simulink model "UPSControl"  (R2025b)
settings: Solver=VariableStepAuto  StartTime=0.0  StopTime=10  FixedStep=Ts  RelTol=1e-3
PostLoadFcn:
  | DataCenterParam;
values from neighbouring files (symbols this model uses):
  generator = struct    [GeneratorParam.m]
  lineInductance = 1e-6    (= 1e-06)    [DataCenterParam.m]    (also in GridParam.m)
  lineResistance = 1e-3    (= 0.001)    [DataCenterParam.m]    (also in GridParam.m)
  loadPower = 5e6    (= 5000000)    [DataCenterParam.m]    (also in LVRT.m; RedundancyAnalysis.m = 10000000)
  machine = struct    [GeneratorParam.m]
  powerTau = 0.005    [DataCenterParam.m]
  Ts = 5e-5    (= 5e-05)    [DataCenterParam.m]    (also in GeneratorParam.m)
  utilizationFactor = 0.45    [DataCenterParam.m]    (also in RedundancyAnalysis.m)
undefined symbols (not defined in the file or in its folder): breaker, ctLimitDelayTime, DiscIntNeverNeededParam, ee_sli_rtmsupport, gcbh, grid, rack, ups
libraries: nesl_utility x96, fl_lib x96, eeGeneralControl x84, ee_lib x80, simulink x68, eeTransforms x30, nesl_utility_internal x16, eeSinusoidalMeasurementV2 x13, slpidlib x12, simulink_extras x12, datacenter_lib x5, batteryecm_lib x4
(part 9 of 13)

== system UPSControl/Server Load/UPS Units/Three UPS Parallel/UPS1/Rectifier/Transfer Control/PCC Voltage Flag ==
  u : Inport
  AND : Logic  IconShape=distinctive  AllPortsSameDT=off  OutDataTypeStr=boolean
  Abs : Abs  SaturateOnIntegerOverflow=off
  Add : Sum  Inputs=+-
  Compare To Constant : simulink/Logic and Bit Operations/Compare To Constant  relop=>  const=0.2  OutDataTypeStr=boolean
  Compare To Constant1 : simulink/Logic and Bit Operations/Compare To Constant  relop=>=  const=0.1  OutDataTypeStr=boolean
  Constant : Constant
  Data Type Conversion : DataTypeConversion  SaturateOnIntegerOverflow=off  RndMeth=Floor
  Data Type Conversion1 : DataTypeConversion  OutDataTypeStr=double  SaturateOnIntegerOverflow=off  RndMeth=Floor
  Discrete-Time Integrator : DiscreteIntegrator  IntegratorMethod=Integration: Backward Euler  ExternalReset=falling  SampleTime=ups.sampleTime  LimitOutput=on  UpperSaturationLimit=0.6  LowerSaturationLimit=0  ICPrevOutput=DiscIntNeverNeededParam  ICPrevScaledInput=DiscIntNeverNeededParam
  VFlag : Outport
  wires:
  AND/1 -> Data Type Conversion/1
  Compare To Constant/1 -> AND/2
  Discrete-Time Integrator/1 -> Compare To Constant/1
  Data Type Conversion/1 -> VFlag/1
  Data Type Conversion1/1 -> Discrete-Time Integrator/1, AND/1, Discrete-Time Integrator/2
  u/1 -> Add/1
  Constant/1 -> Add/2
  Add/1 -> Abs/1
  Compare To Constant1/1 -> Data Type Conversion1/1
  Abs/1 -> Compare To Constant1/1

== system UPSControl/Server Load/UPS Units/Three UPS Parallel/UPS1/Rectifier/Transfer Control/PCC Voltage Flag2 ==
  u : Inport
  AND : Logic  IconShape=distinctive  AllPortsSameDT=off  OutDataTypeStr=boolean
  Abs : Abs  SaturateOnIntegerOverflow=off
  Add : Sum  Inputs=+-
  Compare To Constant : simulink/Logic and Bit Operations/Compare To Constant  relop=>  const=0.15  OutDataTypeStr=boolean
  Compare To Constant1 : simulink/Logic and Bit Operations/Compare To Constant  relop=>=  const=0.9  OutDataTypeStr=boolean
  Constant : Constant
  Data Type Conversion : DataTypeConversion  SaturateOnIntegerOverflow=off  RndMeth=Floor
  Data Type Conversion1 : DataTypeConversion  OutDataTypeStr=double  SaturateOnIntegerOverflow=off  RndMeth=Floor
  Discrete-Time Integrator : DiscreteIntegrator  IntegratorMethod=Integration: Backward Euler  ExternalReset=falling  SampleTime=ups.sampleTime  LimitOutput=on  UpperSaturationLimit=4  LowerSaturationLimit=0  ICPrevOutput=DiscIntNeverNeededParam  ICPrevScaledInput=DiscIntNeverNeededParam
  VFlag : Outport
  wires:
  AND/1 -> Data Type Conversion/1
  Compare To Constant/1 -> AND/2
  Discrete-Time Integrator/1 -> Compare To Constant/1
  Data Type Conversion/1 -> VFlag/1
  Data Type Conversion1/1 -> Discrete-Time Integrator/1, AND/1, Discrete-Time Integrator/2
  u/1 -> Add/1
  Constant/1 -> Add/2
  Add/1 -> Abs/1
  Compare To Constant1/1 -> Data Type Conversion1/1
  Abs/1 -> Compare To Constant1/1

== system UPSControl/Server Load/UPS Units/Three UPS Parallel/UPS1/Rectifier/Transfer Control/PFC Current Flag ==
  u : Inport
  AND : Logic  IconShape=distinctive  AllPortsSameDT=off  OutDataTypeStr=boolean
  Compare To Constant : simulink/Logic and Bit Operations/Compare To Constant  relop=>  const=0.02  OutDataTypeStr=boolean
  Compare To Constant1 : simulink/Logic and Bit Operations/Compare To Constant  relop=<=  const=0.01  OutDataTypeStr=boolean
  Data Type Conversion : DataTypeConversion  SaturateOnIntegerOverflow=off  RndMeth=Floor
  Data Type Conversion1 : DataTypeConversion  OutDataTypeStr=double  SaturateOnIntegerOverflow=off  RndMeth=Floor
  Discrete-Time Integrator : DiscreteIntegrator  IntegratorMethod=Integration: Backward Euler  ExternalReset=falling  SampleTime=ups.sampleTime  LimitOutput=on  UpperSaturationLimit=0.04  LowerSaturationLimit=0  ICPrevOutput=DiscIntNeverNeededParam  ICPrevScaledInput=DiscIntNeverNeededParam
  Scope : Scope  NumInputPorts=2
      settings: ActiveDisplayYMinimum=-1  ActiveDisplayYMaximum=1  DataLoggingVariableName=ScopeData49
  Scope1 : Scope
      settings: ActiveDisplayYMinimum=-1  ActiveDisplayYMaximum=1  DataLoggingVariableName=ScopeData50
  IdFlag : Outport
  wires:
  AND/1 -> Data Type Conversion/1
  Compare To Constant1/1 -> Data Type Conversion1/1
  Compare To Constant/1 -> Scope/2, AND/2
  u/1 -> Compare To Constant1/1
  Discrete-Time Integrator/1 -> Scope1/1, Compare To Constant/1
  Data Type Conversion/1 -> IdFlag/1
  Data Type Conversion1/1 -> Scope/1, Discrete-Time Integrator/1, AND/1, Discrete-Time Integrator/2

== system UPSControl/Server Load/UPS Units/Three UPS Parallel/UPS2/DC-Link/BESS/DC-DC Converter Controller ==
  Voref : Inport
  Vo : Inport  Port=2
  vBatt : Inport  Port=3
  iPFC : Inport  Port=4
  iCharge : Inport  Port=5
  iBatt : Inport  Port=6
  vPCC : Inport  Port=7
  Breaker : Inport  Port=8
  Current Reference Generator : Subsystem
  Gain : Gain  Gain=iBatt
  Mode Control : Subsystem
  Saturation : Saturate  UpperLimit=iBatt  LowerLimit=-iBatt
  Simulink-PS Converter : nesl_utility/Simulink-PS Converter  PhysicalDomain=network_engine_domain  SubClassName=ps_input  LeftPortType=input  RightPortType=output  PseudoPeriodic=off  Frequencies=[]  NoiseDistribution=none  NoiseParameters=[]  Unit=1  AffineConversion=off  FilteringAndDerivatives=provide  SimscapeFilterOrder=1  InputFilterTimeConstant=0.001  UdotUserProvided=0
  Terminator1 : Terminator
  mod : PMIOPort  Side=Right
  wires:
  Gain/1 -> Saturation/1
  iPFC/1 -> Mode Control/1(iPFC)
  vBatt/1 -> Mode Control/3(vBatt)
  Current Reference Generator/1(i) -> Gain/1
  Mode Control/1(DischargeFlag) -> Current Reference Generator/2(DischargeFlag)
  Saturation/1 -> Simulink-PS Converter/1
  iBatt/1 -> Mode Control/7(iBatt)
  vPCC/1 -> Mode Control/4(vPCC)
  Breaker/1 -> Mode Control/5(Breaker)
  iCharge/1 -> Mode Control/6(iCharg)
  Vo/1 -> Mode Control/2(Vdc)
  Mode Control/3(iRef) -> Current Reference Generator/4(I)
  Mode Control/5(Mode) -> Terminator1/1
  Voref/1 -> Current Reference Generator/1(VoRef)
  Mode Control/2(vOut) -> Current Reference Generator/3(Vo)
  Mode Control/4(droopMode) -> Current Reference Generator/5(Mode)
  connections:
  mod/RConn1 -- Simulink-PS Converter/RConn1

== system UPSControl/Server Load/UPS Units/Three UPS Parallel/UPS2/Inverter/Filter & Measurements/PLL & Measurements ==
  V : Inport
  I : Inport  Port=2
  Measurement1 : Subsystem
  Measurement2 : Subsystem
  Subsystem : Subsystem
  Out Bus Element : Outport  PortName=VIbus  Element=Vq
  Out Bus Element1 : Outport  PortName=VIbus  Element=Vd
  Out Bus Element2 : Outport  PortName=VIbus  Element=Freq
  Out Bus Element3 : Outport  PortName=VIbus  Element=Theta
  Out Bus Element4 : Outport  PortName=VIbus  Element=Vmag
  Out Bus Element5 : Outport  PortName=VIbus  Element=Iq
  Out Bus Element6 : Outport  PortName=VIbus  Element=Id
  Out Bus Element7 : Outport  PortName=VIbus  Element=Iabc
  Out Bus Element8 : Outport  PortName=VIbus  Element=Vabc
  wires:
  Subsystem/6(Id1) -> Out Bus Element6/1
  Subsystem/7(Iq1) -> Out Bus Element5/1
  Measurement1/1(Vg) -> Subsystem/2(Iabc), Out Bus Element7/1
  I/1 -> Measurement1/1(u)
  Subsystem/1(mag) -> Out Bus Element4/1
  Measurement2/1(Vg) -> Subsystem/1(Vabc), Out Bus Element8/1
  Subsystem/4(Vd) -> Out Bus Element1/1
  Subsystem/3(angle) -> Out Bus Element3/1
  Subsystem/5(Vq) -> Out Bus Element/1
  Subsystem/2(freq) -> Out Bus Element2/1
  V/1 -> Measurement2/1(u)

== system UPSControl/Server Load/UPS Units/Three UPS Parallel/UPS2/Inverter/Inverter Controller/Current Limiter ==
  BusElementIn : Inport  PortName=VI  Element=Id
  BusElementIn1 : Inport  PortName=VI  Element=Iq
  Vd : Inport  Port=2
  Vq : Inport  Port=3
  Add : Sum  Inputs=+-
  Add1 : Sum  Inputs=+-
  Current Limiter : Subsystem  Variant=on  VariantControlMode=label  VariantControl=Choice  LabelModeActiveChoice=Virtual Impedance
  VdRef : Outport
  VqRef : Outport  Port=2
  Idmax : Outport  Port=3
  Iqmax : Outport  Port=4
  wires:
  BusElementIn/1 -> Current Limiter/1(Igd)
  BusElementIn1/1 -> Current Limiter/2(Igq)
  Current Limiter/3(Idmax) -> Idmax/1
  Current Limiter/4(Iqmax) -> Iqmax/1
  Current Limiter/1(delVd) -> Add/2
  Vd/1 -> Add/1
  Add1/1 -> VqRef/1
  Current Limiter/2(delVq) -> Add1/2
  Vq/1 -> Add1/1
  Add/1 -> VdRef/1

== system UPSControl/Server Load/UPS Units/Three UPS Parallel/UPS2/Inverter/Inverter Controller/Droop Control ==
  note: Frequency difference power
  note: Vs-delV
  BusElementIn : Inport  PortName=Power  Element=activePower
  BusElementIn1 : Inport  PortName=Power  Element=reactivePower
  Add : Sum  Inputs=+-
  Constant1 : Constant  Value=powerFreq*2*pi
  Constant3 : Constant
  Constant4 : Constant  Value=0
  Constant5 : Constant  Value=pi/2
  Gain1 : Gain  Gain=vDroop
  Gain6 : Gain  Gain=fDroop
  Integrator with Wrapped State (Discrete or Continuous) : eeGeneralControl/Integrator with Wrapped State (Discrete or Continuous)  LabelModeActiveChoice=Discrete  WrappedStateUpperValue=2*pi  WrappedStateLowerValue=0  x0=0  Ts=Ts
  Low-Pass Filter (Discrete or Continuous) : eeGeneralControl/Low-Pass Filter (Discrete or Continuous)  K=1  T=0.01  B=inf  A=-inf  init_option=Inherited from block input  x0=0  Ts=-1
  Low-Pass Filter (Discrete or Continuous)1 : eeGeneralControl/Low-Pass Filter (Discrete or Continuous)  K=1  T=0.01  B=inf  A=-inf  init_option=Inherited from block input  x0=0  Ts=-1
  Saturation : Saturate  UpperLimit=1.5  LowerLimit=0.9
  Scope : Scope
      settings: ActiveDisplayYMinimum=1.0057772633115749  ActiveDisplayYMaximum=1.0057796201435223  DataLoggingVariableName=ScopeData3  DataLoggingSaveFormat=Array
  Scope1 : Scope
      settings: ActiveDisplayYMinimum=-1  ActiveDisplayYMaximum=1  DataLoggingVariableName=ScopeData4
  Scope3 : Scope  NumInputPorts=2
      settings: ActiveDisplayYMinimum=-1  ActiveDisplayYMaximum=1  DataLoggingVariableName=ScopeData6  DataLoggingSaveFormat=Array
  Scope4 : Scope  NumInputPorts=2
      settings: ActiveDisplayYMinimum=-1  ActiveDisplayYMaximum=1  DataLoggingVariableName=ScopeData23
  Sum : Sum  Inputs=|++
  Sum1 : Sum  Inputs=|++
  Vdref : Outport
  Vqref : Outport  Port=2
  omega : Outport  Port=3
  Theta : Outport  Port=4
  wires:
  Low-Pass Filter (Discrete or Continuous)/1 -> Gain1/1
  Sum/1 -> Scope4/2, Integrator with Wrapped State (Discrete or Continuous)/1, omega/1
  Gain1/1 -> Sum1/2, Scope3/1
  Sum1/1 -> Scope3/2, Saturation/1  "V"
  Constant5/1 -> Add/2
  Constant3/1 -> Sum1/1
  Saturation/1 -> Scope/1, Vdref/1
  Integrator with Wrapped State (Discrete or Continuous)/1 -> Add/1
  Constant1/1 -> Sum/1
  Add/1 -> Scope1/1, Theta/1
  Gain6/1 -> Scope4/1, Sum/2
  Low-Pass Filter (Discrete or Continuous)1/1 -> Gain6/1
  BusElementIn/1 -> Low-Pass Filter (Discrete or Continuous)1/1
  Constant4/1 -> Vqref/1
  BusElementIn1/1 -> Low-Pass Filter (Discrete or Continuous)/1

== system UPSControl/Server Load/UPS Units/Three UPS Parallel/UPS2/Inverter/Inverter Controller/VoltageCurrentControl ==
  BusElementIn : Inport  PortName=measure  Element=Vq
  BusElementIn1 : Inport  PortName=measure  Element=Vd
  BusElementIn2 : Inport  PortName=measure  Element=Iq
  BusElementIn3 : Inport  PortName=measure  Element=Id
  Vdref : Inport  Port=2
  Vqref : Inport  Port=3
  Idmax : Inport  Port=4
  Iqmax : Inport  Port=5
  w : Inport  Port=6
  Angle : Inport  Port=7
  Controller : Subsystem
  Modulation Signal : Subsystem
  mabc : Outport
  wires:
  Vdref/1 -> Controller/2(Vdref)
  Controller/1(Vd) -> Modulation Signal/1(Vd)
  Modulation Signal/1(mabc) -> mabc/1
  Controller/2(Vq) -> Modulation Signal/2(Vq)
  w/1 -> Controller/1(Angfreq)
  Angle/1 -> Modulation Signal/3(Angle)
  BusElementIn/1 -> Controller/5(Vsq)
  BusElementIn1/1 -> Controller/4(Vsd)
  BusElementIn2/1 -> Controller/7(Iq)
  BusElementIn3/1 -> Controller/6(Id)
  Vqref/1 -> Controller/3(Vqref)
  Idmax/1 -> Controller/8(IqMax)
  Iqmax/1 -> Controller/9(IdMax)

== system UPSControl/Server Load/UPS Units/Three UPS Parallel/UPS2/Rectifier/Filter & AC measurements/Current ==
  Isabc : Inport
  Demux : Demux  Outputs=3
  Mux : Mux  Inputs=3
  Unit Delay : UnitDelay  SampleTime=-1
  Iabc : Outport
  wires:
  Mux/1 -> Iabc/1
  Unit Delay/1 -> Demux/1
  Isabc/1 -> Unit Delay/1
  Demux/1 -> Mux/1
  Demux/2 -> Mux/2
  Demux/3 -> Mux/3

== system UPSControl/Server Load/UPS Units/Three UPS Parallel/UPS2/Rectifier/Filter & AC measurements/PLL ==
  Iabc : Inport
  V : Inport  Port=2
  Constant1 : Constant  Value=pi/2  SampleTime=Ts
  Data Type Conversion Inherited : simulink/Signal Attributes/Data Type Conversion Inherited  ConvertRealWorld=Real World Value  DoSatur=off
  Demux : Demux  Outputs=3
  Park Transform : eeTransforms/Park Transform  AxisAlignment=D-axis  PowerInvariant=off
  "Sinusoidal Measurement (PLL, Three-Phase)" : eeSinusoidalMeasurementV2/Sinusoidal Measurement (PLL, Three-Phase)  InputFilter=on  InputNormalization=off  Kp_LF=ups.AFE.kpPLL  Ki_LF=ups.AFE.kiPLL  F0=frequency  Theta0=0  Ts=Ts
  Sum : Sum  Inputs=|+-
  Terminator : Terminator
  Terminator2 : Terminator
  Id : Outport
  freq : Outport  Port=2
  mag : Outport  Port=3
  wires:
  Data Type Conversion Inherited/1 -> Sum/2
  Constant1/1 -> Data Type Conversion Inherited/2
  V/1 -> "Sinusoidal Measurement (PLL, Three-Phase)"/1
  "Sinusoidal Measurement (PLL, Three-Phase)"/2 -> Sum/1, Data Type Conversion Inherited/1
  Park Transform/1 -> Demux/1
  Demux/3 -> Terminator/1
  Sum/1 -> Park Transform/2
  Demux/1 -> Id/1
  "Sinusoidal Measurement (PLL, Three-Phase)"/1 -> freq/1
  Iabc/1 -> Park Transform/1
  Demux/2 -> Terminator2/1
  "Sinusoidal Measurement (PLL, Three-Phase)"/3 -> mag/1

== system UPSControl/Server Load/UPS Units/Three UPS Parallel/UPS2/Rectifier/Filter & AC measurements/Voltage ==
  Vsabc : Inport
  Demux1 : Demux  Outputs=3
  Mux1 : Mux  Inputs=3
  Unit Delay : UnitDelay  SampleTime=-1
  Vabc : Outport
  wires:
  Mux1/1 -> Vabc/1
  Unit Delay/1 -> Demux1/1
  Vsabc/1 -> Unit Delay/1
  Demux1/1 -> Mux1/1
  Demux1/2 -> Mux1/2
  Demux1/3 -> Mux1/3

== system UPSControl/Server Load/UPS Units/Three UPS Parallel/UPS2/Rectifier/PFC Rectifier Controller/Current Controller ==
  idRef : Inport
  iqRef : Inport  Port=2
  theta : Inport  Port=3
  vd : Inport  Port=4
  vq : Inport  Port=5
  iabc(PU) : Inport  Port=6
  Reset : Inport  Port=7
  Demux1 : Demux  Outputs=3
  Id and Iq Controller : Subsystem
  Inverse Park Transform : eeTransforms/Inverse Park Transform  AxisAlignment=D-axis  PowerInvariant=off
  Park Transform : eeTransforms/Park Transform  AxisAlignment=D-axis  PowerInvariant=off
  Saturation : Saturate  UpperLimit=1.5  LowerLimit=-1.5
  Terminator1 : Terminator
  vabcRef : Outport
  IdCntrlError : Outport  Port=2
  IqCntrlError : Outport  Port=3
  wires:
  Id and Iq Controller/2(IdCntrlError) -> IdCntrlError/1
  Id and Iq Controller/3(IqCntrlError) -> IqCntrlError/1
  Id and Iq Controller/1(vdqoRef) -> Inverse Park Transform/1
  vq/1 -> Id and Iq Controller/6(vq)
  Demux1/2 -> Id and Iq Controller/4(iqSens)  "iqSens"
  iqRef/1 -> Id and Iq Controller/2(iqRef)
  Demux1/1 -> Id and Iq Controller/3(IdSens)  "IdSens"
  idRef/1 -> Id and Iq Controller/1(idRef)
  vd/1 -> Id and Iq Controller/5(vd)
  Inverse Park Transform/1 -> Saturation/1
  iabc(PU)/1 -> Park Transform/1
  theta/1 -> Park Transform/2, Inverse Park Transform/2
  Demux1/3 -> Terminator1/1
  Park Transform/1 -> Demux1/1
  Saturation/1 -> vabcRef/1
  Reset/1 -> Id and Iq Controller/7(Reset)

== system UPSControl/Server Load/UPS Units/Three UPS Parallel/UPS2/Rectifier/PFC Rectifier Controller/DC Voltage Controller and Current Reference ==
  qRef : Inport
  vPeak : Inport  Port=2
  vdcRef : Inport  Port=3
  VdcSens : Inport  Port=4
  Reset : Inport  Port=5
  Constant : Constant  SampleTime=Ts
  Data Type Conversion Inherited : simulink/Signal Attributes/Data Type Conversion Inherited  ConvertRealWorld=Real World Value  DoSatur=off
  Gain : Gain  Gain=-1
  Iq Reference : Subsystem
  Switch : Switch  Criteria=u2 > Threshold  SaturateOnIntegerOverflow=off  InputSameDT=off
  Voltage Controller : Subsystem
  idRef : Outport
  iqRef : Outport  Port=2
  wires:
  Constant/1 -> Data Type Conversion Inherited/2
  Data Type Conversion Inherited/1 -> Switch/3
  Gain/1 -> iqRef/1
  qRef/1 -> Iq Reference/2(Q_ref)
  Voltage Controller/1(Id) -> idRef/1
  vdcRef/1 -> Voltage Controller/1(Vdcref)
  VdcSens/1 -> Voltage Controller/2(Vdcmeas)
  Iq Reference/1(iq_ref) -> Gain/1
  vPeak/1 -> Switch/2, Switch/1, Data Type Conversion Inherited/1
  Switch/1 -> Iq Reference/1(V_mag)
  Reset/1 -> Voltage Controller/3(Reset)

== system UPSControl/Server Load/UPS Units/Three UPS Parallel/UPS2/Rectifier/PFC Rectifier Controller/PLL ==
  V : Inport
  Constant1 : Constant  Value=pi/2  SampleTime=Ts
  Data Type Conversion Inherited : simulink/Signal Attributes/Data Type Conversion Inherited  ConvertRealWorld=Real World Value  DoSatur=off
  Demux : Demux  Outputs=3
  Park Transform : eeTransforms/Park Transform  AxisAlignment=D-axis  PowerInvariant=off
  "Sinusoidal Measurement (PLL, Three-Phase)" : eeSinusoidalMeasurementV2/Sinusoidal Measurement (PLL, Three-Phase)  InputFilter=on  InputNormalization=off  Kp_LF=KpPLL  Ki_LF=KiPLL  F0=Freq  Theta0=0  Ts=Ts
  Sum : Sum  Inputs=|+-
  Terminator : Terminator
  Terminator1 : Terminator
  theta : Outport
  Vd : Outport  Port=2
  Vq : Outport  Port=3
  mag : Outport  Port=4
  wires:
  Data Type Conversion Inherited/1 -> Sum/2
  Constant1/1 -> Data Type Conversion Inherited/2
  V/1 -> Park Transform/1, "Sinusoidal Measurement (PLL, Three-Phase)"/1
  "Sinusoidal Measurement (PLL, Three-Phase)"/2 -> Sum/1, Data Type Conversion Inherited/1
  Park Transform/1 -> Demux/1
  Demux/3 -> Terminator/1
  "Sinusoidal Measurement (PLL, Three-Phase)"/3 -> mag/1
  Sum/1 -> Park Transform/2, theta/1
  Demux/2 -> Vq/1
  Demux/1 -> Vd/1
  "Sinusoidal Measurement (PLL, Three-Phase)"/1 -> Terminator1/1

== system UPSControl/Server Load/UPS Units/Three UPS Parallel/UPS2/Rectifier/Transfer Control/Battery Current Flag ==
  u : Inport
  AND : Logic  IconShape=distinctive  AllPortsSameDT=off  OutDataTypeStr=boolean
  Compare To Constant : simulink/Logic and Bit Operations/Compare To Constant  relop=>=  const=0.04  OutDataTypeStr=boolean
  Compare To Constant1 : simulink/Logic and Bit Operations/Compare To Constant  relop=<=  const=-10  OutDataTypeStr=boolean
  Data Type Conversion : DataTypeConversion  SaturateOnIntegerOverflow=off  RndMeth=Floor
  Data Type Conversion1 : DataTypeConversion  OutDataTypeStr=double  SaturateOnIntegerOverflow=off  RndMeth=Floor
  Discrete-Time Integrator : DiscreteIntegrator  IntegratorMethod=Integration: Backward Euler  ExternalReset=falling  SampleTime=ups.sampleTime  LimitOutput=on  UpperSaturationLimit=0.04  LowerSaturationLimit=0  ICPrevOutput=DiscIntNeverNeededParam  ICPrevScaledInput=DiscIntNeverNeededParam
  Scope : Scope  NumInputPorts=2
      settings: ActiveDisplayYMinimum=-1  ActiveDisplayYMaximum=1  DataLoggingVariableName=ScopeData51
  Scope1 : Scope
      settings: ActiveDisplayYMinimum=-1  ActiveDisplayYMaximum=1  DataLoggingVariableName=ScopeData52
  Scope2 : Scope
      settings: ActiveDisplayYMinimum=-1  ActiveDisplayYMaximum=1  DataLoggingVariableName=ScopeData54
  IBattFlag : Outport
  wires:
  AND/1 -> Data Type Conversion/1
  Compare To Constant1/1 -> Data Type Conversion1/1
  Compare To Constant/1 -> AND/2
  u/1 -> Scope2/1, Compare To Constant1/1
  Discrete-Time Integrator/1 -> Scope/2, Compare To Constant/1
  Data Type Conversion/1 -> Scope1/1, IBattFlag/1
  Data Type Conversion1/1 -> Discrete-Time Integrator/1, Scope/1, AND/1, Discrete-Time Integrator/2

== system UPSControl/Server Load/UPS Units/Three UPS Parallel/UPS2/Rectifier/Transfer Control/Frequency Flag ==
  u : Inport
  AND : Logic  IconShape=distinctive  AllPortsSameDT=off  OutDataTypeStr=boolean
  Abs : Abs  SaturateOnIntegerOverflow=off
  Add : Sum  Inputs=+-
  Compare To Constant : simulink/Logic and Bit Operations/Compare To Constant  relop=>  const=0.5  OutDataTypeStr=boolean
  Compare To Constant1 : simulink/Logic and Bit Operations/Compare To Constant  relop=<=  const=0.01*frequency  OutDataTypeStr=boolean
  Constant : Constant  Value=frequency
  Data Type Conversion : DataTypeConversion  SaturateOnIntegerOverflow=off  RndMeth=Floor
  Data Type Conversion1 : DataTypeConversion  OutDataTypeStr=double  SaturateOnIntegerOverflow=off  RndMeth=Floor
  Discrete-Time Integrator : DiscreteIntegrator  IntegratorMethod=Integration: Backward Euler  ExternalReset=falling  SampleTime=ups.sampleTime  LimitOutput=on  UpperSaturationLimit=0.6  LowerSaturationLimit=0  ICPrevOutput=DiscIntNeverNeededParam  ICPrevScaledInput=DiscIntNeverNeededParam
  FreqFlag : Outport
  wires:
  AND/1 -> Data Type Conversion/1
  Compare To Constant/1 -> AND/2
  Discrete-Time Integrator/1 -> Compare To Constant/1
  Data Type Conversion/1 -> FreqFlag/1
  Data Type Conversion1/1 -> Discrete-Time Integrator/1, AND/1, Discrete-Time Integrator/2
  u/1 -> Add/1
  Constant/1 -> Add/2
  Add/1 -> Abs/1
  Abs/1 -> Compare To Constant1/1
  Compare To Constant1/1 -> Data Type Conversion1/1

== system UPSControl/Server Load/UPS Units/Three UPS Parallel/UPS2/Rectifier/Transfer Control/PCC Voltage Flag ==
  u : Inport
  AND : Logic  IconShape=distinctive  AllPortsSameDT=off  OutDataTypeStr=boolean
  Abs : Abs  SaturateOnIntegerOverflow=off
  Add : Sum  Inputs=+-
  Compare To Constant : simulink/Logic and Bit Operations/Compare To Constant  relop=>  const=0.2  OutDataTypeStr=boolean
  Compare To Constant1 : simulink/Logic and Bit Operations/Compare To Constant  relop=>=  const=0.1  OutDataTypeStr=boolean
  Constant : Constant
  Data Type Conversion : DataTypeConversion  SaturateOnIntegerOverflow=off  RndMeth=Floor
  Data Type Conversion1 : DataTypeConversion  OutDataTypeStr=double  SaturateOnIntegerOverflow=off  RndMeth=Floor
  Discrete-Time Integrator : DiscreteIntegrator  IntegratorMethod=Integration: Backward Euler  ExternalReset=falling  SampleTime=ups.sampleTime  LimitOutput=on  UpperSaturationLimit=0.6  LowerSaturationLimit=0  ICPrevOutput=DiscIntNeverNeededParam  ICPrevScaledInput=DiscIntNeverNeededParam
  VFlag : Outport
  wires:
  AND/1 -> Data Type Conversion/1
  Compare To Constant/1 -> AND/2
  Discrete-Time Integrator/1 -> Compare To Constant/1
  Data Type Conversion/1 -> VFlag/1
  Data Type Conversion1/1 -> Discrete-Time Integrator/1, AND/1, Discrete-Time Integrator/2
  u/1 -> Add/1
  Constant/1 -> Add/2
  Add/1 -> Abs/1
  Compare To Constant1/1 -> Data Type Conversion1/1
  Abs/1 -> Compare To Constant1/1

== system UPSControl/Server Load/UPS Units/Three UPS Parallel/UPS2/Rectifier/Transfer Control/PCC Voltage Flag2 ==
  u : Inport
  AND : Logic  IconShape=distinctive  AllPortsSameDT=off  OutDataTypeStr=boolean
  Abs : Abs  SaturateOnIntegerOverflow=off
  Add : Sum  Inputs=+-
  Compare To Constant : simulink/Logic and Bit Operations/Compare To Constant  relop=>  const=0.15  OutDataTypeStr=boolean
  Compare To Constant1 : simulink/Logic and Bit Operations/Compare To Constant  relop=>=  const=0.9  OutDataTypeStr=boolean
  Constant : Constant
  Data Type Conversion : DataTypeConversion  SaturateOnIntegerOverflow=off  RndMeth=Floor
  Data Type Conversion1 : DataTypeConversion  OutDataTypeStr=double  SaturateOnIntegerOverflow=off  RndMeth=Floor
  Discrete-Time Integrator : DiscreteIntegrator  IntegratorMethod=Integration: Backward Euler  ExternalReset=falling  SampleTime=ups.sampleTime  LimitOutput=on  UpperSaturationLimit=4  LowerSaturationLimit=0  ICPrevOutput=DiscIntNeverNeededParam  ICPrevScaledInput=DiscIntNeverNeededParam
  VFlag : Outport
  wires:
  AND/1 -> Data Type Conversion/1
  Compare To Constant/1 -> AND/2
  Discrete-Time Integrator/1 -> Compare To Constant/1
  Data Type Conversion/1 -> VFlag/1
  Data Type Conversion1/1 -> Discrete-Time Integrator/1, AND/1, Discrete-Time Integrator/2
  u/1 -> Add/1
  Constant/1 -> Add/2
  Add/1 -> Abs/1
  Compare To Constant1/1 -> Data Type Conversion1/1
  Abs/1 -> Compare To Constant1/1

== system UPSControl/Server Load/UPS Units/Three UPS Parallel/UPS2/Rectifier/Transfer Control/PFC Current Flag ==
  u : Inport
  AND : Logic  IconShape=distinctive  AllPortsSameDT=off  OutDataTypeStr=boolean
  Compare To Constant : simulink/Logic and Bit Operations/Compare To Constant  relop=>  const=0.02  OutDataTypeStr=boolean
  Compare To Constant1 : simulink/Logic and Bit Operations/Compare To Constant  relop=<=  const=0.01  OutDataTypeStr=boolean
  Data Type Conversion : DataTypeConversion  SaturateOnIntegerOverflow=off  RndMeth=Floor
  Data Type Conversion1 : DataTypeConversion  OutDataTypeStr=double  SaturateOnIntegerOverflow=off  RndMeth=Floor
  Discrete-Time Integrator : DiscreteIntegrator  IntegratorMethod=Integration: Backward Euler  ExternalReset=falling  SampleTime=ups.sampleTime  LimitOutput=on  UpperSaturationLimit=0.04  LowerSaturationLimit=0  ICPrevOutput=DiscIntNeverNeededParam  ICPrevScaledInput=DiscIntNeverNeededParam
  Scope : Scope  NumInputPorts=2
      settings: ActiveDisplayYMinimum=-1  ActiveDisplayYMaximum=1  DataLoggingVariableName=ScopeData49
  Scope1 : Scope
      settings: ActiveDisplayYMinimum=-1  ActiveDisplayYMaximum=1  DataLoggingVariableName=ScopeData50
  IdFlag : Outport
  wires:
  AND/1 -> Data Type Conversion/1
  Compare To Constant1/1 -> Data Type Conversion1/1
  Compare To Constant/1 -> Scope/2, AND/2
  u/1 -> Compare To Constant1/1
  Discrete-Time Integrator/1 -> Scope1/1, Compare To Constant/1
  Data Type Conversion/1 -> IdFlag/1
  Data Type Conversion1/1 -> Scope/1, Discrete-Time Integrator/1, AND/1, Discrete-Time Integrator/2

== system UPSControl/Server Load/UPS Units/Three UPS Parallel/UPS3/DC-Link/BESS/DC-DC Converter Controller ==
  Voref : Inport
  Vo : Inport  Port=2
  vBatt : Inport  Port=3
  iPFC : Inport  Port=4
  iCharge : Inport  Port=5
  iBatt : Inport  Port=6
  vPCC : Inport  Port=7
  Breaker : Inport  Port=8
  Current Reference Generator : Subsystem
  Gain : Gain  Gain=iBatt
  Mode Control : Subsystem
  Saturation : Saturate  UpperLimit=iBatt  LowerLimit=-iBatt
  Simulink-PS Converter : nesl_utility/Simulink-PS Converter  PhysicalDomain=network_engine_domain  SubClassName=ps_input  LeftPortType=input  RightPortType=output  PseudoPeriodic=off  Frequencies=[]  NoiseDistribution=none  NoiseParameters=[]  Unit=1  AffineConversion=off  FilteringAndDerivatives=provide  SimscapeFilterOrder=1  InputFilterTimeConstant=0.001  UdotUserProvided=0
  Terminator1 : Terminator
  mod : PMIOPort  Side=Right
  wires:
  Gain/1 -> Saturation/1
  iPFC/1 -> Mode Control/1(iPFC)
  vBatt/1 -> Mode Control/3(vBatt)
  Current Reference Generator/1(i) -> Gain/1
  Mode Control/1(DischargeFlag) -> Current Reference Generator/2(DischargeFlag)
  Saturation/1 -> Simulink-PS Converter/1
  iBatt/1 -> Mode Control/7(iBatt)
  vPCC/1 -> Mode Control/4(vPCC)
  Breaker/1 -> Mode Control/5(Breaker)
  iCharge/1 -> Mode Control/6(iCharg)
  Vo/1 -> Mode Control/2(Vdc)
  Mode Control/3(iRef) -> Current Reference Generator/4(I)
  Mode Control/5(Mode) -> Terminator1/1
  Voref/1 -> Current Reference Generator/1(VoRef)
  Mode Control/2(vOut) -> Current Reference Generator/3(Vo)
  Mode Control/4(droopMode) -> Current Reference Generator/5(Mode)
  connections:
  mod/RConn1 -- Simulink-PS Converter/RConn1

== system UPSControl/Server Load/UPS Units/Three UPS Parallel/UPS3/Inverter/Filter & Measurements/PLL & Measurements ==
  V : Inport
  I : Inport  Port=2
  Measurement1 : Subsystem
  Measurement2 : Subsystem
  Subsystem : Subsystem
  Out Bus Element : Outport  PortName=VIbus  Element=Vq
  Out Bus Element1 : Outport  PortName=VIbus  Element=Vd
  Out Bus Element2 : Outport  PortName=VIbus  Element=Freq
  Out Bus Element3 : Outport  PortName=VIbus  Element=Theta
  Out Bus Element4 : Outport  PortName=VIbus  Element=Vmag
  Out Bus Element5 : Outport  PortName=VIbus  Element=Iq
  Out Bus Element6 : Outport  PortName=VIbus  Element=Id
  Out Bus Element7 : Outport  PortName=VIbus  Element=Iabc
  Out Bus Element8 : Outport  PortName=VIbus  Element=Vabc
  wires:
  Subsystem/6(Id1) -> Out Bus Element6/1
  Subsystem/7(Iq1) -> Out Bus Element5/1
  Measurement1/1(Vg) -> Subsystem/2(Iabc), Out Bus Element7/1
  I/1 -> Measurement1/1(u)
  Subsystem/1(mag) -> Out Bus Element4/1
  Measurement2/1(Vg) -> Subsystem/1(Vabc), Out Bus Element8/1
  Subsystem/4(Vd) -> Out Bus Element1/1
  Subsystem/3(angle) -> Out Bus Element3/1
  Subsystem/5(Vq) -> Out Bus Element/1
  Subsystem/2(freq) -> Out Bus Element2/1
  V/1 -> Measurement2/1(u)

== system UPSControl/Server Load/UPS Units/Three UPS Parallel/UPS3/Inverter/Inverter Controller/Current Limiter ==
  BusElementIn : Inport  PortName=VI  Element=Id
  BusElementIn1 : Inport  PortName=VI  Element=Iq
  Vd : Inport  Port=2
  Vq : Inport  Port=3
  Add : Sum  Inputs=+-
  Add1 : Sum  Inputs=+-
  Current Limiter : Subsystem  Variant=on  VariantControlMode=label  VariantControl=Choice  LabelModeActiveChoice=Virtual Impedance
  VdRef : Outport
  VqRef : Outport  Port=2
  Idmax : Outport  Port=3
  Iqmax : Outport  Port=4
  wires:
  BusElementIn/1 -> Current Limiter/1(Igd)
  BusElementIn1/1 -> Current Limiter/2(Igq)
  Current Limiter/3(Idmax) -> Idmax/1
  Current Limiter/4(Iqmax) -> Iqmax/1
  Current Limiter/1(delVd) -> Add/2
  Vd/1 -> Add/1
  Add1/1 -> VqRef/1
  Current Limiter/2(delVq) -> Add1/2
  Vq/1 -> Add1/1
  Add/1 -> VdRef/1

== system UPSControl/Server Load/UPS Units/Three UPS Parallel/UPS3/Inverter/Inverter Controller/Droop Control ==
  note: Frequency difference power
  note: Vs-delV
  BusElementIn : Inport  PortName=Power  Element=activePower
  BusElementIn1 : Inport  PortName=Power  Element=reactivePower
  Add : Sum  Inputs=+-
  Constant1 : Constant  Value=powerFreq*2*pi
  Constant3 : Constant
  Constant4 : Constant  Value=0
  Constant5 : Constant  Value=pi/2
  Gain1 : Gain  Gain=vDroop
  Gain6 : Gain  Gain=fDroop
  Integrator with Wrapped State (Discrete or Continuous) : eeGeneralControl/Integrator with Wrapped State (Discrete or Continuous)  LabelModeActiveChoice=Discrete  WrappedStateUpperValue=2*pi  WrappedStateLowerValue=0  x0=0  Ts=Ts
  Low-Pass Filter (Discrete or Continuous) : eeGeneralControl/Low-Pass Filter (Discrete or Continuous)  K=1  T=0.01  B=inf  A=-inf  init_option=Inherited from block input  x0=0  Ts=-1
  Low-Pass Filter (Discrete or Continuous)1 : eeGeneralControl/Low-Pass Filter (Discrete or Continuous)  K=1  T=0.01  B=inf  A=-inf  init_option=Inherited from block input  x0=0  Ts=-1
  Saturation : Saturate  UpperLimit=1.5  LowerLimit=0.9
  Scope : Scope
      settings: ActiveDisplayYMinimum=1.0057772633115749  ActiveDisplayYMaximum=1.0057796201435223  DataLoggingVariableName=ScopeData3  DataLoggingSaveFormat=Array
  Scope1 : Scope
      settings: ActiveDisplayYMinimum=-1  ActiveDisplayYMaximum=1  DataLoggingVariableName=ScopeData4
  Scope3 : Scope  NumInputPorts=2
      settings: ActiveDisplayYMinimum=-1  ActiveDisplayYMaximum=1  DataLoggingVariableName=ScopeData6  DataLoggingSaveFormat=Array
  Scope4 : Scope  NumInputPorts=2
      settings: ActiveDisplayYMinimum=-1  ActiveDisplayYMaximum=1  DataLoggingVariableName=ScopeData23
  Sum : Sum  Inputs=|++
  Sum1 : Sum  Inputs=|++
  Vdref : Outport
  Vqref : Outport  Port=2
  omega : Outport  Port=3
  Theta : Outport  Port=4
  wires:
  Low-Pass Filter (Discrete or Continuous)/1 -> Gain1/1
  Sum/1 -> Scope4/2, Integrator with Wrapped State (Discrete or Continuous)/1, omega/1
  Gain1/1 -> Sum1/2, Scope3/1
  Sum1/1 -> Scope3/2, Saturation/1  "V"
  Constant5/1 -> Add/2
  Constant3/1 -> Sum1/1
  Saturation/1 -> Scope/1, Vdref/1
  Integrator with Wrapped State (Discrete or Continuous)/1 -> Add/1
  Constant1/1 -> Sum/1
  Add/1 -> Scope1/1, Theta/1
  Gain6/1 -> Scope4/1, Sum/2
  Low-Pass Filter (Discrete or Continuous)1/1 -> Gain6/1
  BusElementIn/1 -> Low-Pass Filter (Discrete or Continuous)1/1
  Constant4/1 -> Vqref/1
  BusElementIn1/1 -> Low-Pass Filter (Discrete or Continuous)/1

== system UPSControl/Server Load/UPS Units/Three UPS Parallel/UPS3/Inverter/Inverter Controller/VoltageCurrentControl ==
  BusElementIn : Inport  PortName=measure  Element=Vq
  BusElementIn1 : Inport  PortName=measure  Element=Vd
  BusElementIn2 : Inport  PortName=measure  Element=Iq
  BusElementIn3 : Inport  PortName=measure  Element=Id
  Vdref : Inport  Port=2
  Vqref : Inport  Port=3
  Idmax : Inport  Port=4
  Iqmax : Inport  Port=5
  w : Inport  Port=6
  Angle : Inport  Port=7
  Controller : Subsystem
  Modulation Signal : Subsystem
  mabc : Outport
  wires:
  Vdref/1 -> Controller/2(Vdref)
  Controller/1(Vd) -> Modulation Signal/1(Vd)
  Modulation Signal/1(mabc) -> mabc/1
  Controller/2(Vq) -> Modulation Signal/2(Vq)
  w/1 -> Controller/1(Angfreq)
  Angle/1 -> Modulation Signal/3(Angle)
  BusElementIn/1 -> Controller/5(Vsq)
  BusElementIn1/1 -> Controller/4(Vsd)
  BusElementIn2/1 -> Controller/7(Iq)
  BusElementIn3/1 -> Controller/6(Id)
  Vqref/1 -> Controller/3(Vqref)
  Idmax/1 -> Controller/8(IqMax)
  Iqmax/1 -> Controller/9(IdMax)

== system UPSControl/Server Load/UPS Units/Three UPS Parallel/UPS3/Rectifier/Filter & AC measurements/Current ==
  Isabc : Inport
  Demux : Demux  Outputs=3
  Mux : Mux  Inputs=3
  Unit Delay : UnitDelay  SampleTime=-1
  Iabc : Outport
  wires:
  Mux/1 -> Iabc/1
  Unit Delay/1 -> Demux/1
  Isabc/1 -> Unit Delay/1
  Demux/1 -> Mux/1
  Demux/2 -> Mux/2
  Demux/3 -> Mux/3

== system UPSControl/Server Load/UPS Units/Three UPS Parallel/UPS3/Rectifier/Filter & AC measurements/PLL ==
  Iabc : Inport
  V : Inport  Port=2
  Constant1 : Constant  Value=pi/2  SampleTime=Ts
  Data Type Conversion Inherited : simulink/Signal Attributes/Data Type Conversion Inherited  ConvertRealWorld=Real World Value  DoSatur=off
  Demux : Demux  Outputs=3
  Park Transform : eeTransforms/Park Transform  AxisAlignment=D-axis  PowerInvariant=off
  "Sinusoidal Measurement (PLL, Three-Phase)" : eeSinusoidalMeasurementV2/Sinusoidal Measurement (PLL, Three-Phase)  InputFilter=on  InputNormalization=off  Kp_LF=ups.AFE.kpPLL  Ki_LF=ups.AFE.kiPLL  F0=frequency  Theta0=0  Ts=Ts
  Sum : Sum  Inputs=|+-
  Terminator : Terminator
  Terminator2 : Terminator
  Id : Outport
  freq : Outport  Port=2
  mag : Outport  Port=3
  wires:
  Data Type Conversion Inherited/1 -> Sum/2
  Constant1/1 -> Data Type Conversion Inherited/2
  V/1 -> "Sinusoidal Measurement (PLL, Three-Phase)"/1
  "Sinusoidal Measurement (PLL, Three-Phase)"/2 -> Sum/1, Data Type Conversion Inherited/1
  Park Transform/1 -> Demux/1
  Demux/3 -> Terminator/1
  Sum/1 -> Park Transform/2
  Demux/1 -> Id/1
  "Sinusoidal Measurement (PLL, Three-Phase)"/1 -> freq/1
  Iabc/1 -> Park Transform/1
  Demux/2 -> Terminator2/1
  "Sinusoidal Measurement (PLL, Three-Phase)"/3 -> mag/1

== system UPSControl/Server Load/UPS Units/Three UPS Parallel/UPS3/Rectifier/Filter & AC measurements/Voltage ==
  Vsabc : Inport
  Demux1 : Demux  Outputs=3
  Mux1 : Mux  Inputs=3
  Unit Delay : UnitDelay  SampleTime=-1
  Vabc : Outport
  wires:
  Mux1/1 -> Vabc/1
  Unit Delay/1 -> Demux1/1
  Vsabc/1 -> Unit Delay/1
  Demux1/1 -> Mux1/1
  Demux1/2 -> Mux1/2
  Demux1/3 -> Mux1/3

== system UPSControl/Server Load/UPS Units/Three UPS Parallel/UPS3/Rectifier/PFC Rectifier Controller/Current Controller ==
  idRef : Inport
  iqRef : Inport  Port=2
  theta : Inport  Port=3
  vd : Inport  Port=4
  vq : Inport  Port=5
  iabc(PU) : Inport  Port=6
  Reset : Inport  Port=7
  Demux1 : Demux  Outputs=3
  Id and Iq Controller : Subsystem
  Inverse Park Transform : eeTransforms/Inverse Park Transform  AxisAlignment=D-axis  PowerInvariant=off
  Park Transform : eeTransforms/Park Transform  AxisAlignment=D-axis  PowerInvariant=off
  Saturation : Saturate  UpperLimit=1.5  LowerLimit=-1.5
  Terminator1 : Terminator
  vabcRef : Outport
  IdCntrlError : Outport  Port=2
  IqCntrlError : Outport  Port=3
  wires:
  Id and Iq Controller/2(IdCntrlError) -> IdCntrlError/1
  Id and Iq Controller/3(IqCntrlError) -> IqCntrlError/1
  Id and Iq Controller/1(vdqoRef) -> Inverse Park Transform/1
  vq/1 -> Id and Iq Controller/6(vq)
  Demux1/2 -> Id and Iq Controller/4(iqSens)  "iqSens"
  iqRef/1 -> Id and Iq Controller/2(iqRef)
  Demux1/1 -> Id and Iq Controller/3(IdSens)  "IdSens"
  idRef/1 -> Id and Iq Controller/1(idRef)
  vd/1 -> Id and Iq Controller/5(vd)
  Inverse Park Transform/1 -> Saturation/1
  iabc(PU)/1 -> Park Transform/1
  theta/1 -> Park Transform/2, Inverse Park Transform/2
  Demux1/3 -> Terminator1/1
  Park Transform/1 -> Demux1/1
  Saturation/1 -> vabcRef/1
  Reset/1 -> Id and Iq Controller/7(Reset)

== system UPSControl/Server Load/UPS Units/Three UPS Parallel/UPS3/Rectifier/PFC Rectifier Controller/DC Voltage Controller and Current Reference ==
  qRef : Inport
  vPeak : Inport  Port=2
  vdcRef : Inport  Port=3
  VdcSens : Inport  Port=4
  Reset : Inport  Port=5
  Constant : Constant  SampleTime=Ts
  Data Type Conversion Inherited : simulink/Signal Attributes/Data Type Conversion Inherited  ConvertRealWorld=Real World Value  DoSatur=off
  Gain : Gain  Gain=-1
  Iq Reference : Subsystem
  Switch : Switch  Criteria=u2 > Threshold  SaturateOnIntegerOverflow=off  InputSameDT=off
  Voltage Controller : Subsystem
  idRef : Outport
  iqRef : Outport  Port=2
  wires:
  Constant/1 -> Data Type Conversion Inherited/2
  Data Type Conversion Inherited/1 -> Switch/3
  Gain/1 -> iqRef/1
  qRef/1 -> Iq Reference/2(Q_ref)
  Voltage Controller/1(Id) -> idRef/1
  vdcRef/1 -> Voltage Controller/1(Vdcref)
  VdcSens/1 -> Voltage Controller/2(Vdcmeas)
  Iq Reference/1(iq_ref) -> Gain/1
  vPeak/1 -> Switch/2, Switch/1, Data Type Conversion Inherited/1
  Switch/1 -> Iq Reference/1(V_mag)
  Reset/1 -> Voltage Controller/3(Reset)

== system UPSControl/Server Load/UPS Units/Three UPS Parallel/UPS3/Rectifier/PFC Rectifier Controller/PLL ==
  V : Inport
  Constant1 : Constant  Value=pi/2  SampleTime=Ts
  Data Type Conversion Inherited : simulink/Signal Attributes/Data Type Conversion Inherited  ConvertRealWorld=Real World Value  DoSatur=off
  Demux : Demux  Outputs=3
  Park Transform : eeTransforms/Park Transform  AxisAlignment=D-axis  PowerInvariant=off
  "Sinusoidal Measurement (PLL, Three-Phase)" : eeSinusoidalMeasurementV2/Sinusoidal Measurement (PLL, Three-Phase)  InputFilter=on  InputNormalization=off  Kp_LF=KpPLL  Ki_LF=KiPLL  F0=Freq  Theta0=0  Ts=Ts
  Sum : Sum  Inputs=|+-
  Terminator : Terminator
  Terminator1 : Terminator
  theta : Outport
  Vd : Outport  Port=2
  Vq : Outport  Port=3
  mag : Outport  Port=4
  wires:
  Data Type Conversion Inherited/1 -> Sum/2
  Constant1/1 -> Data Type Conversion Inherited/2
  V/1 -> Park Transform/1, "Sinusoidal Measurement (PLL, Three-Phase)"/1
  "Sinusoidal Measurement (PLL, Three-Phase)"/2 -> Sum/1, Data Type Conversion Inherited/1
  Park Transform/1 -> Demux/1
  Demux/3 -> Terminator/1
  "Sinusoidal Measurement (PLL, Three-Phase)"/3 -> mag/1
  Sum/1 -> Park Transform/2, theta/1
  Demux/2 -> Vq/1
  Demux/1 -> Vd/1
  "Sinusoidal Measurement (PLL, Three-Phase)"/1 -> Terminator1/1

== system UPSControl/Server Load/UPS Units/Three UPS Parallel/UPS3/Rectifier/Transfer Control/Battery Current Flag ==
  u : Inport
  AND : Logic  IconShape=distinctive  AllPortsSameDT=off  OutDataTypeStr=boolean
  Compare To Constant : simulink/Logic and Bit Operations/Compare To Constant  relop=>=  const=0.04  OutDataTypeStr=boolean
  Compare To Constant1 : simulink/Logic and Bit Operations/Compare To Constant  relop=<=  const=-10  OutDataTypeStr=boolean
  Data Type Conversion : DataTypeConversion  SaturateOnIntegerOverflow=off  RndMeth=Floor
  Data Type Conversion1 : DataTypeConversion  OutDataTypeStr=double  SaturateOnIntegerOverflow=off  RndMeth=Floor
  Discrete-Time Integrator : DiscreteIntegrator  IntegratorMethod=Integration: Backward Euler  ExternalReset=falling  SampleTime=ups.sampleTime  LimitOutput=on  UpperSaturationLimit=0.04  LowerSaturationLimit=0  ICPrevOutput=DiscIntNeverNeededParam  ICPrevScaledInput=DiscIntNeverNeededParam
  Scope : Scope  NumInputPorts=2
      settings: ActiveDisplayYMinimum=-1  ActiveDisplayYMaximum=1  DataLoggingVariableName=ScopeData51
  Scope1 : Scope
      settings: ActiveDisplayYMinimum=-1  ActiveDisplayYMaximum=1  DataLoggingVariableName=ScopeData52
  Scope2 : Scope
      settings: ActiveDisplayYMinimum=-1  ActiveDisplayYMaximum=1  DataLoggingVariableName=ScopeData54
  IBattFlag : Outport
  wires:
  AND/1 -> Data Type Conversion/1
  Compare To Constant1/1 -> Data Type Conversion1/1
  Compare To Constant/1 -> AND/2
  u/1 -> Scope2/1, Compare To Constant1/1
  Discrete-Time Integrator/1 -> Scope/2, Compare To Constant/1
  Data Type Conversion/1 -> Scope1/1, IBattFlag/1
  Data Type Conversion1/1 -> Discrete-Time Integrator/1, Scope/1, AND/1, Discrete-Time Integrator/2

== system UPSControl/Server Load/UPS Units/Three UPS Parallel/UPS3/Rectifier/Transfer Control/Frequency Flag ==
  u : Inport
  AND : Logic  IconShape=distinctive  AllPortsSameDT=off  OutDataTypeStr=boolean
  Abs : Abs  SaturateOnIntegerOverflow=off
  Add : Sum  Inputs=+-
  Compare To Constant : simulink/Logic and Bit Operations/Compare To Constant  relop=>  const=0.5  OutDataTypeStr=boolean
  Compare To Constant1 : simulink/Logic and Bit Operations/Compare To Constant  relop=<=  const=0.01*frequency  OutDataTypeStr=boolean
  Constant : Constant  Value=frequency
  Data Type Conversion : DataTypeConversion  SaturateOnIntegerOverflow=off  RndMeth=Floor
  Data Type Conversion1 : DataTypeConversion  OutDataTypeStr=double  SaturateOnIntegerOverflow=off  RndMeth=Floor
  Discrete-Time Integrator : DiscreteIntegrator  IntegratorMethod=Integration: Backward Euler  ExternalReset=falling  SampleTime=ups.sampleTime  LimitOutput=on  UpperSaturationLimit=0.6  LowerSaturationLimit=0  ICPrevOutput=DiscIntNeverNeededParam  ICPrevScaledInput=DiscIntNeverNeededParam
  FreqFlag : Outport
  wires:
  AND/1 -> Data Type Conversion/1
  Compare To Constant/1 -> AND/2
  Discrete-Time Integrator/1 -> Compare To Constant/1
  Data Type Conversion/1 -> FreqFlag/1
  Data Type Conversion1/1 -> Discrete-Time Integrator/1, AND/1, Discrete-Time Integrator/2
  u/1 -> Add/1
  Constant/1 -> Add/2
  Add/1 -> Abs/1
  Abs/1 -> Compare To Constant1/1
  Compare To Constant1/1 -> Data Type Conversion1/1

== system UPSControl/Server Load/UPS Units/Three UPS Parallel/UPS3/Rectifier/Transfer Control/PCC Voltage Flag ==
  u : Inport
  AND : Logic  IconShape=distinctive  AllPortsSameDT=off  OutDataTypeStr=boolean
  Abs : Abs  SaturateOnIntegerOverflow=off
  Add : Sum  Inputs=+-
  Compare To Constant : simulink/Logic and Bit Operations/Compare To Constant  relop=>  const=0.2  OutDataTypeStr=boolean
  Compare To Constant1 : simulink/Logic and Bit Operations/Compare To Constant  relop=>=  const=0.1  OutDataTypeStr=boolean
  Constant : Constant
  Data Type Conversion : DataTypeConversion  SaturateOnIntegerOverflow=off  RndMeth=Floor
  Data Type Conversion1 : DataTypeConversion  OutDataTypeStr=double  SaturateOnIntegerOverflow=off  RndMeth=Floor
  Discrete-Time Integrator : DiscreteIntegrator  IntegratorMethod=Integration: Backward Euler  ExternalReset=falling  SampleTime=ups.sampleTime  LimitOutput=on  UpperSaturationLimit=0.6  LowerSaturationLimit=0  ICPrevOutput=DiscIntNeverNeededParam  ICPrevScaledInput=DiscIntNeverNeededParam
  VFlag : Outport
  wires:
  AND/1 -> Data Type Conversion/1
  Compare To Constant/1 -> AND/2
  Discrete-Time Integrator/1 -> Compare To Constant/1
  Data Type Conversion/1 -> VFlag/1
  Data Type Conversion1/1 -> Discrete-Time Integrator/1, AND/1, Discrete-Time Integrator/2
  u/1 -> Add/1
  Constant/1 -> Add/2
  Add/1 -> Abs/1
  Compare To Constant1/1 -> Data Type Conversion1/1
  Abs/1 -> Compare To Constant1/1

== system UPSControl/Server Load/UPS Units/Three UPS Parallel/UPS3/Rectifier/Transfer Control/PCC Voltage Flag2 ==
  u : Inport
  AND : Logic  IconShape=distinctive  AllPortsSameDT=off  OutDataTypeStr=boolean
  Abs : Abs  SaturateOnIntegerOverflow=off
  Add : Sum  Inputs=+-
  Compare To Constant : simulink/Logic and Bit Operations/Compare To Constant  relop=>  const=0.15  OutDataTypeStr=boolean
  Compare To Constant1 : simulink/Logic and Bit Operations/Compare To Constant  relop=>=  const=0.9  OutDataTypeStr=boolean
  Constant : Constant
  Data Type Conversion : DataTypeConversion  SaturateOnIntegerOverflow=off  RndMeth=Floor
  Data Type Conversion1 : DataTypeConversion  OutDataTypeStr=double  SaturateOnIntegerOverflow=off  RndMeth=Floor
  Discrete-Time Integrator : DiscreteIntegrator  IntegratorMethod=Integration: Backward Euler  ExternalReset=falling  SampleTime=ups.sampleTime  LimitOutput=on  UpperSaturationLimit=4  LowerSaturationLimit=0  ICPrevOutput=DiscIntNeverNeededParam  ICPrevScaledInput=DiscIntNeverNeededParam
  VFlag : Outport
  wires:
  AND/1 -> Data Type Conversion/1
  Compare To Constant/1 -> AND/2
  Discrete-Time Integrator/1 -> Compare To Constant/1
  Data Type Conversion/1 -> VFlag/1
  Data Type Conversion1/1 -> Discrete-Time Integrator/1, AND/1, Discrete-Time Integrator/2
  u/1 -> Add/1
  Constant/1 -> Add/2
  Add/1 -> Abs/1
  Compare To Constant1/1 -> Data Type Conversion1/1
  Abs/1 -> Compare To Constant1/1

== system UPSControl/Server Load/UPS Units/Three UPS Parallel/UPS3/Rectifier/Transfer Control/PFC Current Flag ==
  u : Inport
  AND : Logic  IconShape=distinctive  AllPortsSameDT=off  OutDataTypeStr=boolean
  Compare To Constant : simulink/Logic and Bit Operations/Compare To Constant  relop=>  const=0.02  OutDataTypeStr=boolean
  Compare To Constant1 : simulink/Logic and Bit Operations/Compare To Constant  relop=<=  const=0.01  OutDataTypeStr=boolean
  Data Type Conversion : DataTypeConversion  SaturateOnIntegerOverflow=off  RndMeth=Floor
  Data Type Conversion1 : DataTypeConversion  OutDataTypeStr=double  SaturateOnIntegerOverflow=off  RndMeth=Floor
  Discrete-Time Integrator : DiscreteIntegrator  IntegratorMethod=Integration: Backward Euler  ExternalReset=falling  SampleTime=ups.sampleTime  LimitOutput=on  UpperSaturationLimit=0.04  LowerSaturationLimit=0  ICPrevOutput=DiscIntNeverNeededParam  ICPrevScaledInput=DiscIntNeverNeededParam
  Scope : Scope  NumInputPorts=2
      settings: ActiveDisplayYMinimum=-1  ActiveDisplayYMaximum=1  DataLoggingVariableName=ScopeData49
  Scope1 : Scope
      settings: ActiveDisplayYMinimum=-1  ActiveDisplayYMaximum=1  DataLoggingVariableName=ScopeData50
  IdFlag : Outport
  wires:
  AND/1 -> Data Type Conversion/1
  Compare To Constant1/1 -> Data Type Conversion1/1
  Compare To Constant/1 -> Scope/2, AND/2
  u/1 -> Compare To Constant1/1
  Discrete-Time Integrator/1 -> Scope1/1, Compare To Constant/1
  Data Type Conversion/1 -> IdFlag/1
  Data Type Conversion1/1 -> Scope/1, Discrete-Time Integrator/1, AND/1, Discrete-Time Integrator/2
